simulink library "bipedlib"  (Simulink 6.1)
values from neighbouring files (symbols this model uses):
  D = [Db1, Db2, Db3, Db4 ... (first row only)    [pdparams.m]
  g = 9.81    [bipedparams.m]
  initstate =     [initstate.mat]
  l1 = 0.5    [bipedparams.m]    (also in pdparams.m = robot.l(2))
  l2 = 0.5    [bipedparams.m]    (also in pdparams.m = robot.l(3))
  P = [Pb1, Pb2, Pb3, Pb4 ... (first row only)    [pdparams.m]
  r0 = l0/2    (= 0.4)    [bipedparams.m]    (also in pdparams.m = robot.r(1))
  ref = [0.04, 0.3261, 0.0314, 0.2199]'    [pdparams.m]
  st = 0.005    [bipedparams.m]    (also in pdparams.m)
undefined symbols (not defined in the file or in its folder): dataprop, groundp, initswitch, knees, robot
libraries: bipedlib x11, simulink x6, crclib x1
(part 2 of 2)

== system bipedlib/Biped model/Knee stopper/Knee control (L)/PD ==
  Position : Inport  Orientation=left  Port=1  LatchInput=off
  Speed : Inport  Orientation=left  Port=2  LatchInput=off
  Enable : EnablePort
  Constant : Constant  Orientation=left  Value=kneemin
  Gain : Gain  Orientation=left  Gain=kk  SaturateOnIntegerOverflow=on
  Gain1 : Gain  Orientation=left  Gain=bk  SaturateOnIntegerOverflow=on
  Saturation : Saturate  Orientation=left  UpperLimit=inf  LowerLimit=0
  Sum : Sum  Orientation=left  Inputs=+-|  SaturateOnIntegerOverflow=on
  Sum2 : Sum  Orientation=left  Inputs=|+-  SaturateOnIntegerOverflow=on
  Moment : Outport  Orientation=left  OutputWhenDisabled=reset  InitialOutput=0
  wires:
  Position/1 -> Sum/2
  Speed/1 -> Gain1/1
  Gain1/1 -> Sum2/2
  Gain/1 -> Sum2/1
  Sum2/1 -> Saturation/1
  Sum/1 -> Gain/1
  Constant/1 -> Sum/1
  Saturation/1 -> Moment/1

== system bipedlib/Biped model/Knee stopper/Knee control (L)/PD1 ==
  Position : Inport  Orientation=left  Port=1  LatchInput=off
  Speed : Inport  Orientation=left  Port=2  LatchInput=off
  Enable : EnablePort
  Constant : Constant  Orientation=left  Value=kneemax
  Gain : Gain  Orientation=left  Gain=kk  SaturateOnIntegerOverflow=on
  Gain1 : Gain  Orientation=left  Gain=bk  SaturateOnIntegerOverflow=on
  Saturation : Saturate  Orientation=left  UpperLimit=0  LowerLimit=-inf
  Sum : Sum  Orientation=left  Inputs=+-|  SaturateOnIntegerOverflow=on
  Sum2 : Sum  Orientation=left  Inputs=|+-  SaturateOnIntegerOverflow=on
  Moment : Outport  Orientation=left  OutputWhenDisabled=reset  InitialOutput=0
  wires:
  Saturation/1 -> Moment/1
  Constant/1 -> Sum/1
  Sum/1 -> Gain/1
  Sum2/1 -> Saturation/1
  Gain/1 -> Sum2/1
  Gain1/1 -> Sum2/2
  Speed/1 -> Gain1/1
  Position/1 -> Sum/2

== system bipedlib/PD control/Controller/PDs/Discrete PD1 ==
  In : Inport  Port=1  LatchInput=off
  P : Inport  Port=2  LatchInput=off
  D : Inport  Port=3  LatchInput=off
  Gain5 : Gain  Gain=1/st  SaturateOnIntegerOverflow=on
  Product : Product  SaturateOnIntegerOverflow=on
  Product1 : Product  Inputs=3  SaturateOnIntegerOverflow=on
  Relational Operator : RelationalOperator  Operator===
  Sum : Sum  SaturateOnIntegerOverflow=on
  Sum2 : Sum  Inputs=-+|  SaturateOnIntegerOverflow=on  InputSameDT=on
  Unit Delay : UnitDelay  SampleTime=-1
  Unit Delay2 : UnitDelay  SampleTime=-1
  Out : Outport
  wires:
  Product/1 -> Sum/1
  In/1 -> Sum2/2, Unit Delay/1, Product/2
  Unit Delay/1 -> Sum2/1
  Gain5/1 -> Sum/2
  Sum/1 -> Out/1
  Sum2/1 -> Product1/1
  Product1/1 -> Gain5/1
  D/1 -> Product1/2, Unit Delay2/1, Relational Operator/1
  Unit Delay2/1 -> Relational Operator/2
  Relational Operator/1 -> Product1/3
  P/1 -> Product/1

== system bipedlib/PD control/Create references/Walking cycle/Both edges to impulse ==
  In1 : Inport  Port=1  LatchInput=off
  Logical Operator1 : Logic  Operator=NOT  AllPortsSameDT=off
  Relational Operator : RelationalOperator  Operator=~=
  Unit Delay : UnitDelay  X0=1  SampleTime=st
  Out1 : Outport
  wires:
  In1/1 -> Relational Operator/1, Unit Delay/1
  Unit Delay/1 -> Relational Operator/2
  Relational Operator/1 -> Logical Operator1/1
  Logical Operator1/1 -> Out1/1

== system bipedlib/PD control/Create references/Walking cycle/Double support phase control ==
  note: 0.118
  Old ref : Inport  Port=1  LatchInput=off
  State : Inport  Port=2  LatchInput=off
  Enable : EnablePort  StatesWhenEnabling=reset
  Constant : Constant  Value=0.1
  Reference changes : Subsystem
  Relational Operator1 : RelationalOperator  Operator=<=
  Selector : Selector  InputPortWidth=9
  Sum : Sum  SaturateOnIntegerOverflow=on
  Sum2 : Sum  Inputs=+-  SaturateOnIntegerOverflow=on
  leg position : Fcn  Expr=u(1) - r0*sin(u(3)) - l1*sin(u(3)-u(5)) - l2*sin(u(3)-u(5)+u(7))
  New ref : Outport
  wires:
  Old ref/1 -> Sum/1
  Sum/1 -> New ref/1
  State/1 -> Selector/1, leg position/1
  leg position/1 -> Sum2/1  "xrg"
  Selector/1 -> Sum2/2  "x0"
  Relational Operator1/1 -> Reference changes/Enable
  Sum2/1 -> Relational Operator1/1
  Constant/1 -> Relational Operator1/2
  Reference changes/1(Out) -> Sum/2

== system bipedlib/PD control/Create references/Walking cycle/No support control ==
  Old ref : Inport  Port=1  LatchInput=off
  Enable : EnablePort
  New ref : Outport
  wires:
  Old ref/1 -> New ref/1

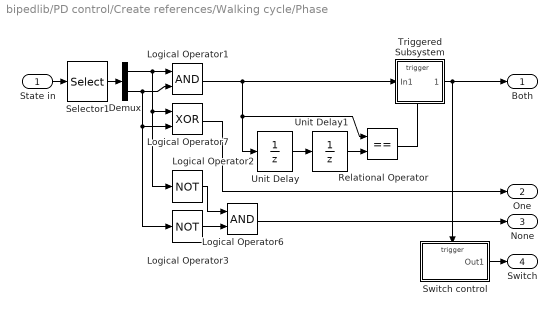
== system bipedlib/PD control/Create references/Walking cycle/Phase ==
  State in : Inport  Port=1  LatchInput=off
  Demux : Demux  Outputs=2
  Logical Operator1 : Logic  AllPortsSameDT=off
  Logical Operator2 : Logic  Operator=NOT  AllPortsSameDT=off
  Logical Operator3 : Logic  Operator=NOT  AllPortsSameDT=off
  Logical Operator6 : Logic  AllPortsSameDT=off
  Logical Operator7 : Logic  Operator=XOR  AllPortsSameDT=off
  Relational Operator : RelationalOperator  Operator===
  Selector1 : Selector  Elements=[8,9]  InputPortWidth=9
  Switch control : Subsystem  TreatAsAtomicUnit=on
  Triggered Subsystem : Subsystem  TreatAsAtomicUnit=on
  Unit Delay : UnitDelay  X0=1  SampleTime=st
  Unit Delay1 : UnitDelay  X0=1  SampleTime=st
  Both : Outport
  One : Outport  Port=2
  None : Outport  Port=3
  Switch : Outport  Port=4
  wires:
  State in/1 -> Selector1/1
  Selector1/1 -> Demux/1
  Switch control/1(Out1) -> Switch/1
  Demux/1 -> Logical Operator1/1, Logical Operator7/1, Logical Operator2/1
  Demux/2 -> Logical Operator1/2, Logical Operator7/2, Logical Operator3/1
  Logical Operator1/1 -> Unit Delay/1, Relational Operator/1, Triggered Subsystem/1(In1)
  Logical Operator7/1 -> One/1
  Logical Operator6/1 -> None/1
  Unit Delay/1 -> Unit Delay1/1
  Relational Operator/1 -> Triggered Subsystem/Trigger
  Triggered Subsystem/1(Out1) -> Both/1, Switch control/Trigger
  Unit Delay1/1 -> Relational Operator/2
  Logical Operator2/1 -> Logical Operator6/1
  Logical Operator3/1 -> Logical Operator6/2

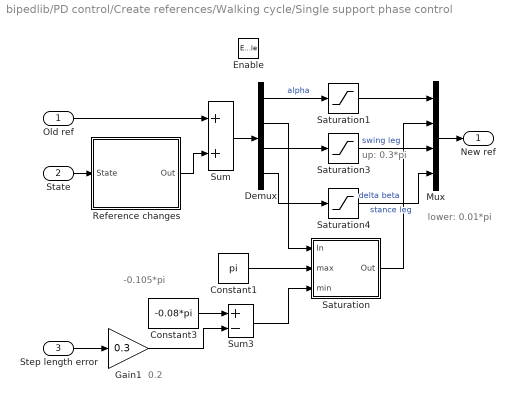
== system bipedlib/PD control/Create references/Walking cycle/Single support phase control ==
  note: up: 0.3*pi
  note: 0.2
  note: lower: 0.01*pi
  note: -0.105*pi
  Old ref : Inport  Port=1  LatchInput=off
  State : Inport  Port=2  LatchInput=off
  Step length error : Inport  Port=3  LatchInput=off
  Enable : EnablePort  StatesWhenEnabling=reset
  Constant1 : Constant  Value=pi
  Constant3 : Constant  Value=-0.08*pi
  Demux : Demux
  Gain1 : Gain  Gain=0.3  SaturateOnIntegerOverflow=on
  Mux : Mux
  Reference changes : Subsystem
  Saturation : Subsystem
  Saturation1 : Saturate  UpperLimit=pi/2  LowerLimit=-pi/2  LinearizeAsGain=off
  Saturation3 : Saturate  UpperLimit=0.2*pi  LowerLimit=0.07*pi  LinearizeAsGain=off
  Saturation4 : Saturate  UpperLimit=pi  LowerLimit=0.015*pi  LinearizeAsGain=off
  Sum : Sum  SaturateOnIntegerOverflow=on
  Sum3 : Sum  Inputs=+-  SaturateOnIntegerOverflow=on
  New ref : Outport
  wires:
  Sum/1 -> Demux/1
  Old ref/1 -> Sum/1
  State/1 -> Reference changes/1(State)
  Step length error/1 -> Gain1/1
  Mux/1 -> New ref/1
  Demux/2 -> Saturation/1(In)
  Saturation/1(Out) -> Mux/2  "delta beta"
  Constant1/1 -> Saturation/2(max)
  Demux/1 -> Saturation1/1  "alpha"
  Demux/3 -> Saturation3/1
  Saturation3/1 -> Mux/3  "swing leg"
  Demux/4 -> Saturation4/1
  Saturation4/1 -> Mux/4  "stance leg"
  Constant3/1 -> Sum3/1
  Gain1/1 -> Sum3/2
  Sum3/1 -> Saturation/3(min)
  Reference changes/1(Out) -> Sum/2
  Saturation1/1 -> Mux/1

== system bipedlib/PD control/Create references/Walking cycle/Step length error ==
  note: 0.335
  State : Inport  Port=1  LatchInput=off
  Trigger : TriggerPort
  Constant : Constant  Value=0.352
  Leg tip positions : Subsystem
  Sum : Sum  Inputs=-+  SaturateOnIntegerOverflow=on
  Sum1 : Sum  Inputs=-+  SaturateOnIntegerOverflow=on
  Error : Outport  InitialOutput=0
  wires:
  State/1 -> Leg tip positions/1(In1)
  Leg tip positions/2(xrg) -> Sum/2
  Leg tip positions/1(xlg) -> Sum/1
  Sum/1 -> Sum1/2
  Sum1/1 -> Error/1
  Constant/1 -> Sum1/1

== system bipedlib/PD control/Create references/Walking cycle/Switch legs ==
  State : Inport  Port=1  LatchInput=off
  Switch : Inport  Port=2  LatchInput=off
  Selector : Selector  Elements=[1, 2, 3, 5, 4, 7, 6, 9, 8]  InputPortWidth=9
  Switch1 : Switch  Threshold=1  SaturateOnIntegerOverflow=on
  Out : Outport
  wires:
  Switch/1 -> Switch1/2
  State/1 -> Switch1/1, Selector/1
  Selector/1 -> Switch1/3
  Switch1/1 -> Out/1

== system bipedlib/Biped model/Ground contact/Calculate forces (L)/Controls/Control x'g ==
  Sensor : Inport  Orientation=left  Port=1  LatchInput=off
  Position : Inport  Orientation=left  Port=2  LatchInput=off
  Speed : Inport  Orientation=left  Port=3  LatchInput=off
  Normal force : Inport  Orientation=left  Port=4  LatchInput=off
  Control : Subsystem  Orientation=left
  Data Type Conversion : DataTypeConversion  Orientation=left  SaturateOnIntegerOverflow=on  RndMeth=Zero
  Logical Operator : Logic  Orientation=left  Operator=OR  AllPortsSameDT=off
  Memory : Memory  X0=gcstate(2)  InheritSampleTime=on
  Mux2 : Mux  Orientation=left  Inputs=2
  Rising edge to impulse : Subsystem  Orientation=left
  Update initial position : Subsystem  Orientation=left  TreatAsAtomicUnit=on
  Force : Outport  Orientation=left
  gcstate : Outport  Orientation=left  Port=2
  wires:
  Memory/1 -> Control/5(Prev sliding), Data Type Conversion/1, Logical Operator/2
  Position/1 -> Control/1(Position), Update initial position/1(In1)
  Speed/1 -> Control/3(Speed)
  Control/1(Force) -> Force/1
  Normal force/1 -> Control/4(Normal force)
  Control/2(Sliding) -> Memory/1
  Sensor/1 -> Control/Enable, Rising edge to impulse/1(In1)
  Logical Operator/1 -> Update initial position/Enable
  Rising edge to impulse/1(Out1) -> Logical Operator/1
  Update initial position/1(Out1) -> Control/2(Initial position), Mux2/1
  Data Type Conversion/1 -> Mux2/2
  Mux2/1 -> gcstate/1

== system bipedlib/Biped model/Ground contact/Calculate forces (L)/Controls/Control y'g ==
  Position : Inport  Orientation=left  Port=1  LatchInput=off
  Speed : Inport  Orientation=left  Port=2  LatchInput=off
  Ground level : Constant  Orientation=left  Value=0
  PD : Subsystem  Orientation=left  TreatAsAtomicUnit=on
  Relational Operator : RelationalOperator  Orientation=left  Operator=<  LogicOutDataTypeMode=Boolean
  Force : Outport  Orientation=left
  Sensor : Outport  Orientation=left  Port=2
  wires:
  Ground level/1 -> Relational Operator/2
  PD/1(Force) -> Force/1
  Position/1 -> Relational Operator/1, PD/1(Position)
  Speed/1 -> PD/2(Speed)
  Relational Operator/1 -> PD/Enable, Sensor/1

== system bipedlib/Biped model/Ground contact/Calculate forces (L)/Leg tip projection/Projection ==
  xy : Inport  Orientation=left  Port=1  LatchInput=off
  Tangential : Inport  Orientation=left  Port=2  LatchInput=off
  Normal : Inport  Orientation=left  Port=3  LatchInput=off
  Origo : Inport  Orientation=left  Port=4  LatchInput=off
  Dot product : Subsystem  Orientation=left
  Dot product1 : bipedlib/Biped model/Ground contact/Calculate forces (L)/Leg tip projection/Projection/Dot product  Orientation=left  SimViewingDevice=off  DataTypeOverride=UseLocalSettings  MinMaxOverflowLogging=UseLocalSettings
      settings: Permissions=ReadWrite  RTWFcnNameOpts=Auto  RTWFileNameOpts=Auto
  Sum : Sum  Orientation=left  Inputs=+-  SaturateOnIntegerOverflow=on
  xtan : Outport  Orientation=left
  ynorm : Outport  Orientation=left  Port=2
  wires:
  Tangential/1 -> Dot product/2(In2)
  xy/1 -> Sum/1
  Origo/1 -> Sum/2
  Sum/1 -> Dot product/1(In1), Dot product1/1
  Dot product/1(Out1) -> xtan/1
  Dot product1/1 -> ynorm/1
  Normal/1 -> Dot product1/2

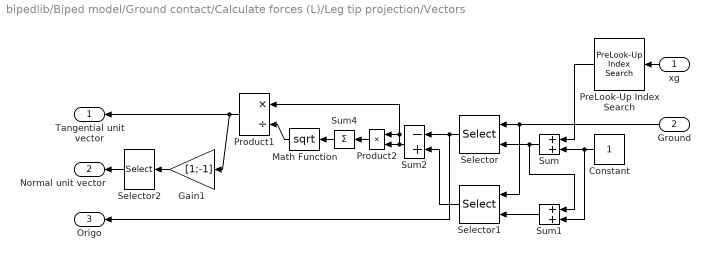
== system bipedlib/Biped model/Ground contact/Calculate forces (L)/Leg tip projection/Vectors ==
  xg : Inport  Orientation=left  Port=1  LatchInput=off
  Ground : Inport  Orientation=left  Port=2  LatchInput=off
  Constant : Constant  Orientation=left
  Gain1 : Gain  Orientation=left  Gain=[1;-1]  SaturateOnIntegerOverflow=on
  Math Function : Math  Orientation=left  Operator=sqrt  SaturateOnIntegerOverflow=on
  PreLook-Up Index Search : simulink/Look-Up Tables/PreLook-Up Index Search  Orientation=left  bpData=ground(1,:)  searchMode=Linear Search  cacheBpFlag=on  outputFlag=on  extrapMode=Clip to Range  rangeErrorMode=None
  Product1 : Product  Orientation=left  Inputs=*/  SaturateOnIntegerOverflow=on
  Product2 : Product  Orientation=left  SaturateOnIntegerOverflow=on
  Selector : Selector  Orientation=left  InputType=Matrix  ElementSrc=External  Elements=[1 3]  Rows=-1  ColumnSrc=External  InputPortWidth=3
  Selector1 : Selector  Orientation=left  InputType=Matrix  ElementSrc=External  Elements=[1 3]  Rows=-1  ColumnSrc=External  InputPortWidth=3
  Selector2 : Selector  Orientation=left  Elements=[2,1]  InputPortWidth=2
  Sum : Sum  Orientation=left  SaturateOnIntegerOverflow=on
  Sum1 : Sum  Orientation=left  SaturateOnIntegerOverflow=on
  Sum2 : Sum  Orientation=left  Inputs=-+  SaturateOnIntegerOverflow=on
  Sum4 : Sum  Orientation=left  Inputs=+  SaturateOnIntegerOverflow=on
  Tangential unit vector : Outport  Orientation=left
  Normal unit vector : Outport  Orientation=left  Port=2
  Origo : Outport  Orientation=left  Port=3
  wires:
  Ground/1 -> Selector/1, Selector1/1
  Math Function/1 -> Product1/2
  Sum2/1 -> Product1/1, Product2/1, Product2/2
  Selector/1 -> Sum2/1, Origo/1
  Selector1/1 -> Sum2/2
  Sum1/1 -> Selector1/2
  Selector2/1 -> Normal unit vector/1
  Product1/1 -> Tangential unit vector/1, Gain1/1
  xg/1 -> PreLook-Up Index Search/1
  PreLook-Up Index Search/1 -> Sum/1
  Gain1/1 -> Selector2/1
  Sum/1 -> Selector/2, Sum1/1
  Constant/1 -> Sum/2, Sum1/2
  Sum4/1 -> Math Function/1
  Product2/1 -> Sum4/1

== system bipedlib/PD control/Create references/Walking cycle/Double support phase control/Reference changes ==
  note: 0.04
  note: -0.05
  Enable : EnablePort
  Ground : Ground
  Mux : Mux
  bend knee : Constant  Value=0.01
  decrease db : Constant  Value=-0.001
  Out : Outport  OutputWhenDisabled=reset  InitialOutput=0
  wires:
  Ground/1 -> Mux/4, Mux/1
  bend knee/1 -> Mux/3  "rear leg knee"
  Mux/1 -> Out/1
  decrease db/1 -> Mux/2  "delta beta"

== system bipedlib/PD control/Create references/Walking cycle/Phase/Switch control ==
  note: 0 = right leg swings,
      | 1 = left leg swings
  Trigger : TriggerPort
  Logical Operator : Logic  Operator=NOT  AllPortsSameDT=off
  Unit Delay : UnitDelay  Orientation=left  X0=1  SampleTime=-1
  Out1 : Outport  InitialOutput=1
  wires:
  Unit Delay/1 -> Logical Operator/1
  Logical Operator/1 -> Out1/1, Unit Delay/1

== system bipedlib/PD control/Create references/Walking cycle/Phase/Triggered Subsystem ==
  In1 : Inport  Port=1  LatchInput=off
  Trigger : TriggerPort
  Out1 : Outport  InitialOutput=1
  wires:
  In1/1 -> Out1/1

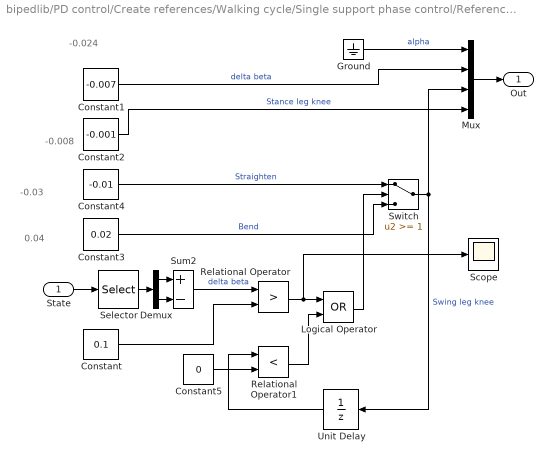
== system bipedlib/PD control/Create references/Walking cycle/Single support phase control/Reference changes ==
  note: -0.03
  note: -0.024
  note: 0.04
  note: -0.008
  State : Inport  Port=1  LatchInput=off
  Constant : Constant  Value=0.1
  Constant1 : Constant  Value=-0.007
  Constant2 : Constant  Value=-0.001
  Constant3 : Constant  Value=0.02
  Constant4 : Constant  Value=-0.01
  Constant5 : Constant  Value=0
  Demux : Demux  Outputs=2
  Ground : Ground
  Logical Operator : Logic  Operator=OR  AllPortsSameDT=off
  Mux : Mux
  Relational Operator : RelationalOperator  Operator=>
  Relational Operator1 : RelationalOperator  Operator=<
  Scope : Scope
      settings: SaveName=ScopeData2
  Selector : Selector  Elements=[4, 5]  InputPortWidth=9
  Sum2 : Sum  Inputs=+-  SaturateOnIntegerOverflow=on
  Switch : Switch  Threshold=1  SaturateOnIntegerOverflow=on
  Unit Delay : UnitDelay  Orientation=left  X0=0.04  SampleTime=st
  Out : Outport  InitialOutput=0
  wires:
  Constant2/1 -> Mux/4  "Stance leg knee"
  Constant3/1 -> Switch/3  "Bend"
  Constant4/1 -> Switch/1  "Straighten"
  State/1 -> Selector/1
  Selector/1 -> Demux/1
  Demux/1 -> Sum2/1
  Demux/2 -> Sum2/2
  Sum2/1 -> Relational Operator/1  "delta beta"
  Mux/1 -> Out/1
  Constant/1 -> Relational Operator/2
  Constant1/1 -> Mux/2  "delta beta"
  Ground/1 -> Mux/1  "alpha"
  Unit Delay/1 -> Relational Operator1/1
  Relational Operator1/1 -> Logical Operator/2
  Constant5/1 -> Relational Operator1/2
  Relational Operator/1 -> Scope/1, Logical Operator/1
  Logical Operator/1 -> Switch/2
  Switch/1 -> Mux/3, Unit Delay/1  "Swing leg knee"

== system bipedlib/PD control/Create references/Walking cycle/Single support phase control/Saturation ==
  In : Inport  Port=1  LatchInput=off
  max : Inport  Port=2  LatchInput=off
  min : Inport  Port=3  LatchInput=off
  Relational Operator : RelationalOperator  Operator=<
  Relational Operator1 : RelationalOperator  Operator=>
  Switch : Switch  Threshold=1  SaturateOnIntegerOverflow=on
  Switch1 : Switch  Threshold=1  SaturateOnIntegerOverflow=on
  Out : Outport
  wires:
  In/1 -> Switch/1, Relational Operator/1
  max/1 -> Relational Operator/2, Switch/3
  min/1 -> Relational Operator1/2, Switch1/3
  Relational Operator/1 -> Switch/2
  Switch/1 -> Relational Operator1/1, Switch1/1
  Relational Operator1/1 -> Switch1/2
  Switch1/1 -> Out/1

== system bipedlib/PD control/Create references/Walking cycle/Step length error/Leg tip positions ==
  In1 : Inport  Orientation=down  Port=1  LatchInput=off
  Fcn : Fcn  Expr=u(1) - r0*sin(u(3)) - l1*sin(u(3)-u(4)) - l2*sin(u(3)-u(4)+u(6))
  Fcn2 : Fcn  Expr=u(1) - r0*sin(u(3)) - l1*sin(u(3)-u(5)) - l2*sin(u(3)-u(5)+u(7))
  xlg : Outport
  xrg : Outport  Port=2
  wires:
  In1/1 -> Fcn/1, Fcn2/1
  Fcn/1 -> xlg/1
  Fcn2/1 -> xrg/1

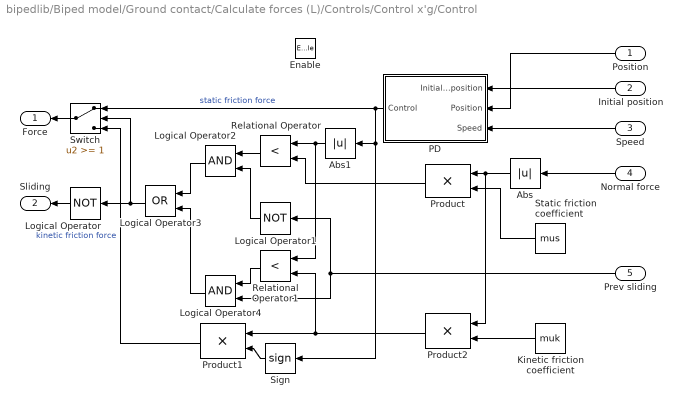
== system bipedlib/Biped model/Ground contact/Calculate forces (L)/Controls/Control x'g/Control ==
  Position : Inport  Orientation=left  Port=1  LatchInput=off
  Initial position : Inport  Orientation=left  Port=2  LatchInput=off
  Speed : Inport  Orientation=left  Port=3  LatchInput=off
  Normal force : Inport  Orientation=left  Port=4  LatchInput=off
  Prev sliding : Inport  Orientation=left  Port=5  LatchInput=off
  Enable : EnablePort
  Abs : Abs  Orientation=left  SaturateOnIntegerOverflow=on
  Abs1 : Abs  Orientation=left  SaturateOnIntegerOverflow=on
  Kinetic friction coefficient : Constant  Orientation=left  Value=muk
  Logical Operator : Logic  Orientation=left  Operator=NOT  AllPortsSameDT=off
  Logical Operator1 : Logic  Orientation=left  Operator=NOT  AllPortsSameDT=off
  Logical Operator2 : Logic  Orientation=left  AllPortsSameDT=off
  Logical Operator3 : Logic  Orientation=left  Operator=OR  AllPortsSameDT=off
  Logical Operator4 : Logic  Orientation=left  AllPortsSameDT=off
  PD : Subsystem  Orientation=left
  Product : Product  Orientation=left  SaturateOnIntegerOverflow=on
  Product1 : Product  Orientation=left  SaturateOnIntegerOverflow=on
  Product2 : Product  Orientation=left  SaturateOnIntegerOverflow=on
  Relational Operator : RelationalOperator  Orientation=left  Operator=<
  Relational Operator1 : RelationalOperator  Orientation=left  Operator=<
  Sign : Signum  Orientation=left
  Static friction coefficient : Constant  Orientation=left  Value=mus
  Switch : Switch  Orientation=left  Threshold=1  SaturateOnIntegerOverflow=on
  Force : Outport  Orientation=left  OutputWhenDisabled=reset  InitialOutput=0
  Sliding : Outport  Orientation=left  Port=2  OutputWhenDisabled=reset  InitialOutput=0
  wires:
  Position/1 -> PD/2(Position)
  Initial position/1 -> PD/1(Initial position)
  Speed/1 -> PD/3(Speed)
  PD/1(Control) -> Abs1/1, Sign/1, Switch/1  "static friction force"
  Switch/1 -> Force/1
  Normal force/1 -> Abs/1
  Static friction coefficient/1 -> Product/2
  Product/1 -> Relational Operator/2
  Kinetic friction coefficient/1 -> Product2/2
  Product1/1 -> Switch/3  "kinetic friction force"
  Logical Operator/1 -> Sliding/1
  Abs/1 -> Product/1, Product2/1
  Abs1/1 -> Relational Operator/1, Relational Operator1/1
  Prev sliding/1 -> Logical Operator1/1, Logical Operator4/2
  Relational Operator/1 -> Logical Operator2/1
  Logical Operator1/1 -> Logical Operator2/2
  Logical Operator3/1 -> Switch/2, Logical Operator/1
  Logical Operator2/1 -> Logical Operator3/1
  Logical Operator4/1 -> Logical Operator3/2
  Relational Operator1/1 -> Logical Operator4/1
  Product2/1 -> Product1/1, Relational Operator1/2
  Sign/1 -> Product1/2

== system bipedlib/Biped model/Ground contact/Calculate forces (L)/Controls/Control x'g/Rising edge to impulse ==
  In1 : Inport  Orientation=left  Port=1  LatchInput=off
  Memory : Memory  Orientation=left
  Relational Operator : RelationalOperator  Orientation=left  Operator=>
  Out1 : Outport  Orientation=left
  wires:
  In1/1 -> Memory/1, Relational Operator/1
  Memory/1 -> Relational Operator/2
  Relational Operator/1 -> Out1/1

== system bipedlib/Biped model/Ground contact/Calculate forces (L)/Controls/Control x'g/Update initial position ==
  In1 : Inport  Port=1  LatchInput=off
  Enable : EnablePort
  Out1 : Outport  InitialOutput=gcstate(1)
  wires:
  In1/1 -> Out1/1

== system bipedlib/Biped model/Ground contact/Calculate forces (L)/Controls/Control y'g/PD ==
  Position : Inport  Orientation=left  Port=1  LatchInput=off
  Speed : Inport  Orientation=left  Port=2  LatchInput=off
  Enable : EnablePort
  Constant : Constant  Orientation=left  Value=0
  Gain : Gain  Orientation=left  Gain=ky  SaturateOnIntegerOverflow=on
  Gain1 : Gain  Orientation=left  Gain=by  SaturateOnIntegerOverflow=on
  Saturation : Saturate  Orientation=left  UpperLimit=inf  LowerLimit=0  ZeroCross=off
  Sum : Sum  Orientation=left  Inputs=+-|  SaturateOnIntegerOverflow=on
  Sum2 : Sum  Orientation=left  Inputs=|+-  SaturateOnIntegerOverflow=on
  Force : Outport  Orientation=left  OutputWhenDisabled=reset  InitialOutput=0
  wires:
  Position/1 -> Sum/2
  Constant/1 -> Sum/1
  Sum/1 -> Gain/1
  Speed/1 -> Gain1/1
  Gain/1 -> Sum2/1
  Gain1/1 -> Sum2/2
  Sum2/1 -> Saturation/1
  Saturation/1 -> Force/1

== system bipedlib/Biped model/Ground contact/Calculate forces (L)/Leg tip projection/Projection/Dot product ==
  In1 : Inport  Orientation=left  Port=1  LatchInput=off
  In2 : Inport  Orientation=left  Port=2  LatchInput=off
  Product : Product  Orientation=left  SaturateOnIntegerOverflow=on
  Sum1 : Sum  Orientation=left  Inputs=+  SaturateOnIntegerOverflow=on
  Out1 : Outport  Orientation=left
  wires:
  Product/1 -> Sum1/1
  In1/1 -> Product/1
  Sum1/1 -> Out1/1
  In2/1 -> Product/2

== system bipedlib/Biped model/Ground contact/Calculate forces (L)/Controls/Control x'g/Control/PD ==
  Initial position : Inport  Orientation=left  Port=1  LatchInput=off
  Position : Inport  Orientation=left  Port=2  LatchInput=off
  Speed : Inport  Orientation=left  Port=3  LatchInput=off
  Gain : Gain  Orientation=left  Gain=kx  SaturateOnIntegerOverflow=on
  Gain1 : Gain  Orientation=left  Gain=bx  SaturateOnIntegerOverflow=on
  Sum : Sum  Orientation=left  Inputs=+-|  SaturateOnIntegerOverflow=on
  Sum2 : Sum  Orientation=left  Inputs=|+-  SaturateOnIntegerOverflow=on
  Control : Outport  Orientation=left
  wires:
  Sum/1 -> Gain/1
  Gain1/1 -> Sum2/2
  Gain/1 -> Sum2/1
  Initial position/1 -> Sum/1
  Position/1 -> Sum/2
  Sum2/1 -> Control/1
  Speed/1 -> Gain1/1
